simulink model "opv_receiver_HDL_coder_input_constructed_MSK"  (R2023a)
settings: Solver=FixedStepDiscrete  StartTime=0.0  StopTime=0.01*(samples_per_frame/sample_rate)  RelTol=1e-3
values from neighbouring files (symbols this model uses):
  bits_per_symbol = 2    [opv.m]
  carrier_frequency = carrier_frequency_multiple_ceil*(orthogonal_frequency)    [opv.m]
  compFilt = design(compSpec,'SystemObject',true)    [opv.m]
  device_clock = 245.76e6    (= 245760000)    [opv.m]
  finalFilt = design(finalSpec,'equiripple','SystemObject',true)    [opv.m]
  intermediateFilt = design(intermediateSpec,'equiripple','SystemObject',true)    [opv.m]
  orthogonal_frequency = 1/(4*bit_period)    (= 13550)    [opv.m]
  symbol_rate = 27100    [opv.m]
libraries: dsphdlfiltering2 x8, dspsrcs4 x4, commrandsrc3 x2, dsphdlsigops2 x2, dspfdesign x1
(part 1 of 4)
settings Model: Creator=matt  LastModifiedBy=matt
settings OptimizationCC: BlockReduction=off  ConditionallyExecuteInputs=off  DefaultParameterBehavior=Inlined
settings DebuggingCC: AlgebraicLoopMsg=error
settings HardwareCC: ProdBitPerPointer=32  ProdBitPerSizeT=32  ProdBitPerPtrDiffT=32  ProdLargestAtomicFloat=None  ProdIntDivRoundTo=Undefined  ProdEndianess=Unspecified  ProdWordSize=32  ProdHWDeviceType=ASIC/FPGA->ASIC/FPGA  TargetBitPerLong=64  TargetBitPerPointer=64  TargetBitPerSizeT=64  TargetBitPerPtrDiffT=64  TargetLongLongMode=on  TargetIntDivRoundTo=Zero  TargetEndianess=LittleEndian  TargetWordSize=64  TargetHWDeviceType=Custom Processor->MATLAB Host Computer  ProdEqTarget=off

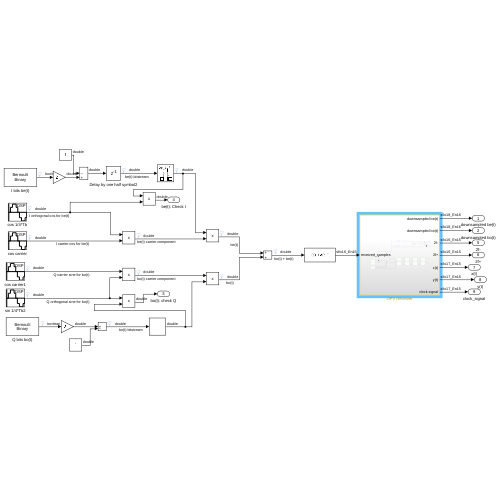
[thumbnail: Simulink's stored preview of the top-level diagram]
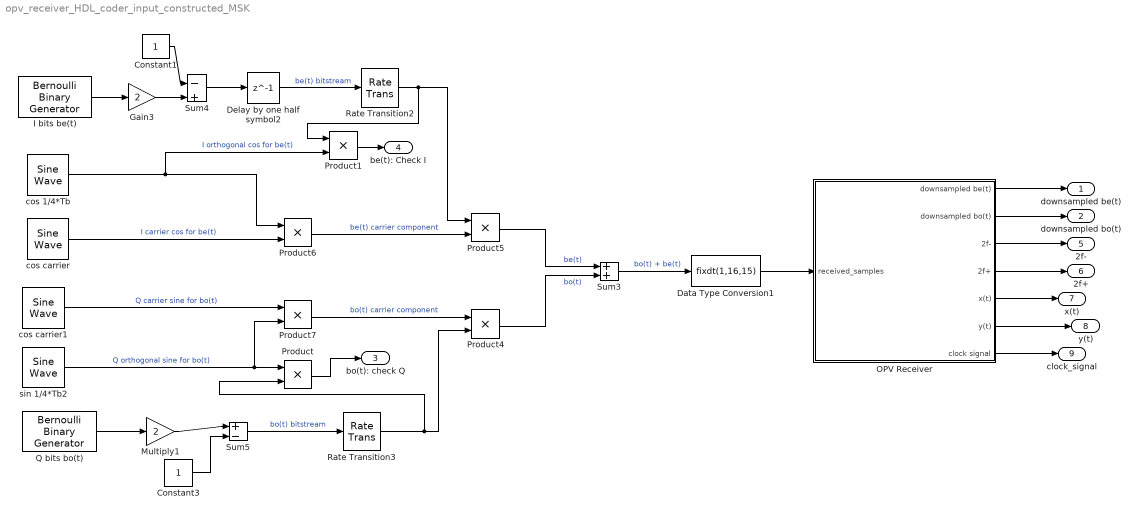
== system opv_receiver_HDL_coder_input_constructed_MSK ==
  Constant1 : Constant  OutDataTypeStr=double  SampleTime=1/symbol_rate
  Constant3 : Constant  OutDataTypeStr=double  SampleTime=1/symbol_rate
  Data Type Conversion1 : DataTypeConversion  OutDataTypeStr=fixdt(1,16,15)  SaturateOnIntegerOverflow=off  RndMeth=Floor
  Delay by one half symbol2 : Delay  DelayLength=1  SampleTime=1/(bits_per_symbol*symbol_rate)
  Gain3 : Gain  Gain=2  OutDataTypeStr=double
  I bits be(t) : commrandsrc3/Bernoulli Binary Generator  ProbabilityOfZero=0.5  SeedSource=Auto  Seed=0  SampleTime=1/(symbol_rate)  SamplesPerFrame=1  OutputDataType=boolean  SimulateUsing=Interpreted execution
  Multiply1 : Gain  Gain=2  OutDataTypeStr=double
  OPV Receiver : Subsystem  TreatAsAtomicUnit=on
      settings: LibrarySourceBlock=|
      | hdlsllib/Ports &
      | Subsystems/Subsystem
  Product{,1,4..5} (4 alike) : Product
  Product6 : Product  OutDataTypeStr=double
  Product7 : Product  OutDataTypeStr=double
  Q bits bo(t) : commrandsrc3/Bernoulli Binary Generator  ProbabilityOfZero=0.5  SeedSource=Auto  Seed=0  SampleTime=1/(symbol_rate)  SamplesPerFrame=1  OutputDataType=boolean  SimulateUsing=Interpreted execution
  Rate Transition2 : RateTransition  Deterministic=off  OutPortSampleTimeMultiple=device_clock/symbol_rate  OutPortSampleTime=1/device_clock
  Rate Transition3 : RateTransition  Deterministic=off  OutPortSampleTimeMultiple=device_clock/symbol_rate  OutPortSampleTime=1/device_clock
  Sum3 : Sum  AccumDataTypeStr=double
  Sum4 : Sum  Inputs=|-+  AccumDataTypeStr=double
  Sum5 : Sum  Inputs=|+-  AccumDataTypeStr=double
  cos 1/4*Tb : dspsrcs4/Sine Wave  Amplitude=1  Frequency=orthogonal_frequency  Phase=pi/2  SampleMode=Discrete  OutComplex=Real  CompMethod=Trigonometric fcn  TableSize=Speed  SampleTime=1/device_clock  SamplesPerFrame=1  ResetState=Restart at time zero  OutputFrames=off  dataType=double  wordLen=16  udDataType=sfix(16)  fracBitsMode=User-defined  numFracBits=0  OutDataTypeStr=double  LastOutDataTypeStr=double
  cos carrier : dspsrcs4/Sine Wave  Amplitude=1  Frequency=carrier_frequency  Phase=pi/2  SampleMode=Discrete  OutComplex=Real  CompMethod=Trigonometric fcn  TableSize=Speed  SampleTime=1/device_clock  SamplesPerFrame=1  ResetState=Restart at time zero  OutputFrames=off  dataType=double  wordLen=16  udDataType=sfix(16)  fracBitsMode=User-defined  numFracBits=0  OutDataTypeStr=double  LastOutDataTypeStr=double
  cos carrier1 : dspsrcs4/Sine Wave  Amplitude=1  Frequency=carrier_frequency  Phase=0  SampleMode=Discrete  OutComplex=Real  CompMethod=Trigonometric fcn  TableSize=Speed  SampleTime=1/device_clock  SamplesPerFrame=1  ResetState=Restart at time zero  OutputFrames=off  dataType=double  wordLen=16  udDataType=sfix(16)  fracBitsMode=User-defined  numFracBits=0  OutDataTypeStr=double  LastOutDataTypeStr=double
  sin 1/4*Tb2 : dspsrcs4/Sine Wave  Amplitude=1  Frequency=orthogonal_frequency  Phase=0  SampleMode=Discrete  OutComplex=Real  CompMethod=Trigonometric fcn  TableSize=Speed  SampleTime=1/device_clock  SamplesPerFrame=1  ResetState=Restart at time zero  OutputFrames=off  dataType=double  wordLen=16  udDataType=sfix(16)  fracBitsMode=User-defined  numFracBits=0  OutDataTypeStr=double  LastOutDataTypeStr=double
  downsampled be(t) : Outport
  downsampled bo(t) : Outport  Port=2
  bo(t): check Q : Outport  Port=3
  be(t): Check I : Outport  Port=4
  2f- : Outport  Port=5
  2f+ : Outport  Port=6
  x(t) : Outport  Port=7
  y(t) : Outport  Port=8
  clock_signal : Outport  Port=9
  wires:
  OPV Receiver/1(downsampled be(t)) -> downsampled be(t)/1
  OPV Receiver/2(downsampled bo(t)) -> downsampled bo(t)/1
  sin 1/4*Tb2/1 -> Product7/2, Product/1  "Q orthogonal sine for bo(t)"
  cos carrier1/1 -> Product7/1  "Q carrier sine for bo(t)"
  Sum3/1 -> Data Type Conversion1/1  "bo(t) + be(t)"
  Product6/1 -> Product5/2  "be(t) carrier component"
  Product7/1 -> Product4/1  "bo(t) carrier component"
  cos 1/4*Tb/1 -> Product6/1, Product1/2  "I orthogonal cos for be(t)"
  cos carrier/1 -> Product6/2  "I carrier cos for be(t)"
  Data Type Conversion1/1 -> OPV Receiver/1(received_samples)
  Q bits bo(t)/1 -> Multiply1/1
  Multiply1/1 -> Sum5/1
  Constant3/1 -> Sum5/2
  I bits be(t)/1 -> Gain3/1
  Product4/1 -> Sum3/2  "bo(t)"
  Product5/1 -> Sum3/1  "be(t)"
  Sum4/1 -> Delay by one half symbol2/1
  Rate Transition2/1 -> Product5/1, Product1/1
  Rate Transition3/1 -> Product/2, Product4/2
  Sum5/1 -> Rate Transition3/1  "bo(t) bitstream"
  Gain3/1 -> Sum4/2
  Constant1/1 -> Sum4/1
  Product/1 -> bo(t): check Q/1
  Product1/1 -> be(t): Check I/1
  Delay by one half symbol2/1 -> Rate Transition2/1  "be(t) bitstream"
  OPV Receiver/3(2f-) -> 2f-/1
  OPV Receiver/4(2f+) -> 2f+/1
  OPV Receiver/5(x(t)) -> x(t)/1
  OPV Receiver/6(y(t)) -> y(t)/1
  OPV Receiver/7(clock signal) -> clock_signal/1

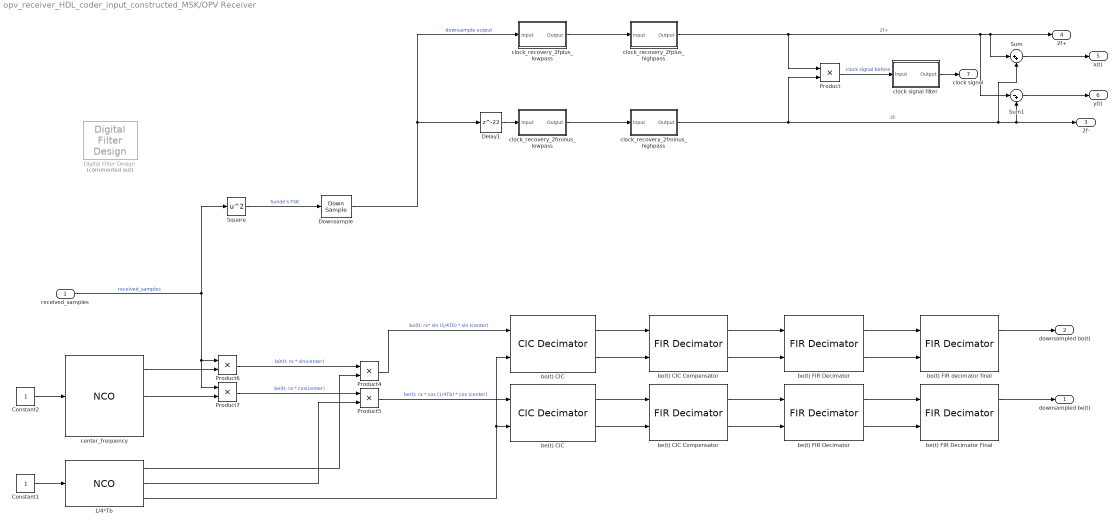
== system opv_receiver_HDL_coder_input_constructed_MSK/OPV Receiver ==
  received_samples : Inport
  " 1/4*Tb" : dsphdlsigops2/NCO  PhaseIncrementSource=Property  PhaseIncrement=phase_increment_bo_be  PhaseOffsetSource=Property  PhaseOffset=0  DitherSource=Property  NumDitherBits=16  SamplesPerFrame=1  LUTCompress=off  ResetAction=off  Waveform=Sine and cosine  PhasePort=off  SimulateUsing=Code generation  AccumulatorWL=32  PhaseQuantization=on  NumQuantizerAccumulatorBits=12  OutputDataType=Binary point scaling  OutputWL=16  OutputFL=15
      settings: LibrarySourceBlock=dsphdlsrcs2/NCO
  Constant1 : Constant  OutDataTypeStr=boolean  SampleTime=1/(device_clock)
  Constant2 : Constant  OutDataTypeStr=boolean  SampleTime=1/(device_clock)
  Delay1 : Delay  DelayLength=22
  Digital Filter Design : dspfdesign/Digital Filter Design  Commented=on  mwdsp_browser_bugfix_var=off
  Downsample : DownSample  N=128  RateOptions=Allow multirate processing
  Product : Product
  Product{4..7} (4 alike) : Product  OutDataTypeStr=fixdt(1,16,15)
  Square : Math  Operator=square  SignedPower=on  RndMeth=Zero
  Sum : Sum  Inputs=|++
  Sum1 : Sum  Inputs=|-+
  be(t) CIC : dsphdlfiltering2/CIC Decimator  DecimationSource=Property  DecimationFactor=cicParams.DecimationFactor  MaxDecimationFactor=2  DifferentialDelay=cicParams.DifferentialDelay  NumSections=cicParams.NumSections  GainCorrection=on  SimulateUsing=Code generation  OutputDataType=Minimum section word lengths  OutputWordLength=18  ResetInputPort=off  HDLGlobalReset=off
  be(t) CIC Compensator : dsphdlfiltering2/FIR Decimator  Numerator=compFilt.Numerator  FilterStructure=Direct form systolic  DecimationFactor=2  NumCycles=2  SimulateUsing=Code generation  roundingMode=Floor  overflowMode=off  CoefficientsDataTypeStr=Inherit: Same word length as input  OutputDataTypeStr=fixdt(1,18,16)  ResetInputPort=off  HDLGlobalReset=off
  be(t) FIR Decimator : dsphdlfiltering2/FIR Decimator  Numerator=intermediateFilt.Numerator  FilterStructure=Direct form systolic  DecimationFactor=4  NumCycles=8  SimulateUsing=Code generation  roundingMode=Floor  overflowMode=off  CoefficientsDataTypeStr=Inherit: Same word length as input  OutputDataTypeStr=fixdt(1,18,16)  ResetInputPort=off  HDLGlobalReset=off
  be(t) FIR Decimator Final : dsphdlfiltering2/FIR Decimator  Numerator=finalFilt.Numerator  FilterStructure=Direct form systolic  DecimationFactor=4  NumCycles=16  SimulateUsing=Code generation  roundingMode=Floor  overflowMode=off  CoefficientsDataTypeStr=Inherit: Same word length as input  OutputDataTypeStr=fixdt(1,18,16)  ResetInputPort=off  HDLGlobalReset=off
  bo(t) CIC : dsphdlfiltering2/CIC Decimator  DecimationSource=Property  DecimationFactor=cicParams.DecimationFactor  MaxDecimationFactor=2  DifferentialDelay=cicParams.DifferentialDelay  NumSections=cicParams.NumSections  GainCorrection=on  SimulateUsing=Code generation  OutputDataType=Minimum section word lengths  OutputWordLength=18  ResetInputPort=off  HDLGlobalReset=off
  bo(t) CIC Compensator : dsphdlfiltering2/FIR Decimator  Numerator=compFilt.Numerator  FilterStructure=Direct form systolic  DecimationFactor=2  NumCycles=2  SimulateUsing=Code generation  roundingMode=Floor  overflowMode=off  CoefficientsDataTypeStr=Inherit: Same word length as input  OutputDataTypeStr=fixdt(1,18,16)  ResetInputPort=off  HDLGlobalReset=off
  bo(t) FIR Decimator : dsphdlfiltering2/FIR Decimator  Numerator=intermediateFilt.Numerator  FilterStructure=Direct form systolic  DecimationFactor=4  NumCycles=8  SimulateUsing=Code generation  roundingMode=Floor  overflowMode=off  CoefficientsDataTypeStr=Inherit: Same word length as input  OutputDataTypeStr=fixdt(1,18,16)  ResetInputPort=off  HDLGlobalReset=off
  bo(t) FIR decimator final : dsphdlfiltering2/FIR Decimator  Numerator=finalFilt.Numerator  FilterStructure=Direct form systolic  DecimationFactor=4  NumCycles=16  SimulateUsing=Code generation  roundingMode=Floor  overflowMode=off  CoefficientsDataTypeStr=Inherit: Same word length as input  OutputDataTypeStr=fixdt(1,18,16)  ResetInputPort=off  HDLGlobalReset=off
  center_frequency : dsphdlsigops2/NCO  PhaseIncrementSource=Property  PhaseIncrement=phase_increment_carrier  PhaseOffsetSource=Property  PhaseOffset=0  DitherSource=Property  NumDitherBits=16  SamplesPerFrame=1  LUTCompress=off  ResetAction=off  Waveform=Sine and cosine  PhasePort=off  SimulateUsing=Code generation  AccumulatorWL=32  PhaseQuantization=on  NumQuantizerAccumulatorBits=12  OutputDataType=Binary point scaling  OutputWL=16  OutputFL=15
      settings: LibrarySourceBlock=dsphdlsrcs2/NCO
  clock signal filter : Subsystem  Tag=FilterWizardSubSystem
      settings: ErrorFcn=dspFilterRealizedInBasicElemsAlgLoopErrFcnCallback
  clock_recovery_2fminus_highpass : Subsystem  Tag=FilterWizardSubSystem
      settings: ErrorFcn=dspFilterRealizedInBasicElemsAlgLoopErrFcnCallback
  clock_recovery_2fminus_lowpass : Subsystem  Tag=FilterWizardSubSystem
      settings: ErrorFcn=dspFilterRealizedInBasicElemsAlgLoopErrFcnCallback
  clock_recovery_2fplus_highpass : Subsystem  Tag=FilterWizardSubSystem
      settings: ErrorFcn=dspFilterRealizedInBasicElemsAlgLoopErrFcnCallback
  clock_recovery_2fplus_lowpass : Subsystem  Tag=FilterWizardSubSystem
      settings: ErrorFcn=dspFilterRealizedInBasicElemsAlgLoopErrFcnCallback
  downsampled be(t) : Outport
  downsampled bo(t) : Outport  Port=2
  2f- : Outport  Port=3
  2f+ : Outport  Port=4
  x(t) : Outport  Port=5
  y(t) : Outport  Port=6
  clock signal : Outport  Port=7
  wires:
  Product5/1 -> be(t) CIC/1  "be(t): rx * cos (1/4Tb) * cos (center)"
  Product6/1 -> Product4/1  "b0(t): rx * sin(center)"
  Constant2/1 -> center_frequency/1
  Constant1/1 -> " 1/4*Tb"/1
  Product7/1 -> Product5/1  "be(t): rx * cos(center)"
  Product4/1 -> bo(t) CIC/1  "bo(t): rx* sin (1/4Tb) * sin (center)"
  " 1/4*Tb"/1 -> Product4/2
  " 1/4*Tb"/3 -> bo(t) CIC/2, be(t) CIC/2
  received_samples/1 -> Square/1, Product7/1, Product6/1  "received_samples"
  be(t) CIC Compensator/1 -> be(t) FIR Decimator/1
  be(t) CIC Compensator/2 -> be(t) FIR Decimator/2
  be(t) CIC/1 -> be(t) CIC Compensator/1
  be(t) CIC/2 -> be(t) CIC Compensator/2
  bo(t) CIC Compensator/1 -> bo(t) FIR Decimator/1
  bo(t) CIC Compensator/2 -> bo(t) FIR Decimator/2
  bo(t) CIC/1 -> bo(t) CIC Compensator/1
  bo(t) CIC/2 -> bo(t) CIC Compensator/2
  be(t) FIR Decimator/2 -> be(t) FIR Decimator Final/2
  be(t) FIR Decimator/1 -> be(t) FIR Decimator Final/1
  bo(t) FIR Decimator/2 -> bo(t) FIR decimator final/2
  bo(t) FIR Decimator/1 -> bo(t) FIR decimator final/1
  be(t) FIR Decimator Final/1 -> downsampled be(t)/1
  bo(t) FIR decimator final/1 -> downsampled bo(t)/1
  center_frequency/1 -> Product6/2
  center_frequency/2 -> Product7/2
  " 1/4*Tb"/2 -> Product5/2
  clock_recovery_2fminus_lowpass/1(Output) -> clock_recovery_2fminus_highpass/1(Input)
  Square/1 -> Downsample/1  "Sunde's FSK"
  clock_recovery_2fplus_lowpass/1(Output) -> clock_recovery_2fplus_highpass/1(Input)
  Downsample/1 -> clock_recovery_2fplus_lowpass/1(Input), Delay1/1  "downsample output"
  clock_recovery_2fminus_highpass/1(Output) -> Product/2, Sum/2, Sum1/2, 2f-/1  "2f-"
  Sum/1 -> x(t)/1
  Sum1/1 -> y(t)/1
  Product/1 -> clock signal filter/1(Input)  "clock signal before"
  clock_recovery_2fplus_highpass/1(Output) -> Product/1, Sum1/1, Sum/1, 2f+/1  "2f+"
  clock signal filter/1(Output) -> clock signal/1
  Delay1/1 -> clock_recovery_2fminus_lowpass/1(Input)
